simulink model "HallEffect"  (R2024b)
settings: Solver=FixedStepAuto  StartTime=0.0  StopTime=inf  FixedStep=0.01  RelTol=1e-3  EnableMultiTasking=on
libraries: stm32f4xxblockslib x1, simulink x1, dspstat3 x1
settings Model: STM32="{\"AnalogInput\":[{\"ID\":\"untitled:1\"},{\"ID\":\"HallEffect:1\"}]}"  Creator=jirat  LastModifiedBy=jirat
settings OptimizationCC: DefaultParameterBehavior=Inlined  EnhancedBackFolding=on  PassReuseOutputArgsAs=Individual arguments  ZeroExternalMemoryAtStartup=off  ZeroInternalMemoryAtStartup=off  MaxStackSize=512  OptimizeBlockOrder=speed  DifferentSizesBufferReuse=on  OptimizationCustomize=off  EfficientTunableParamExpr=on
settings DebuggingCC: ParameterTunabilityLossMsg=error
settings HardwareCC: ProdBitPerPointer=32  ProdBitPerSizeT=32  ProdBitPerPtrDiffT=32  ProdLargestAtomicInteger=Long  ProdLargestAtomicFloat=Double  ProdWordSize=32  ProdLongLongMode=on  ProdHWDeviceType=ARM Compatible->ARM Cortex-M
settings SFSimCC: MATLABDynamicMemAlloc=off
settings RTWCC: Description=Embedded Coder  SystemTargetFile=ert.tlc  HardwareBoard=STM32G4xx Based  TemplateMakefile=ert_default_tmf  Toolchain=GNU Tools for ARM Embedded Processors
settings CodeAppCC: ForceParamTrailComments=on  IgnoreCustomStorageClasses=off  OperatorAnnotations=on  SimulinkDataObjDesc=on  SFDataObjDesc=on  InsertBlockDesc=on
settings ERTTargetCC: TargetLangStandard=C99 (ISO)  CodeReplacementLibrary=ARM Cortex-M  ExtModeTransport=3  ExtModeStaticAlloc=on  ExtModeStaticAllocSize=2048  ExtModeMexFile=ext_xcp  ExtModeIntrfLevel=Level2 - Open

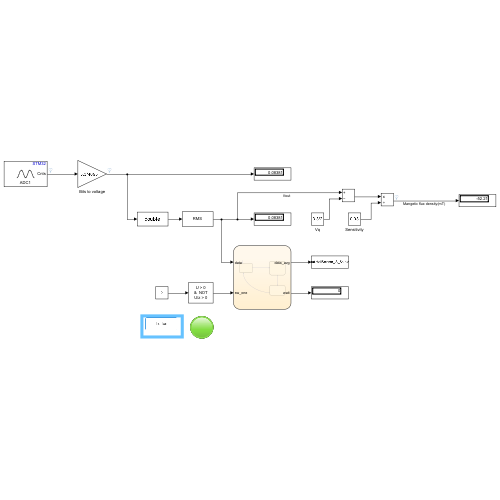
[thumbnail: Simulink's stored preview of the top-level diagram]
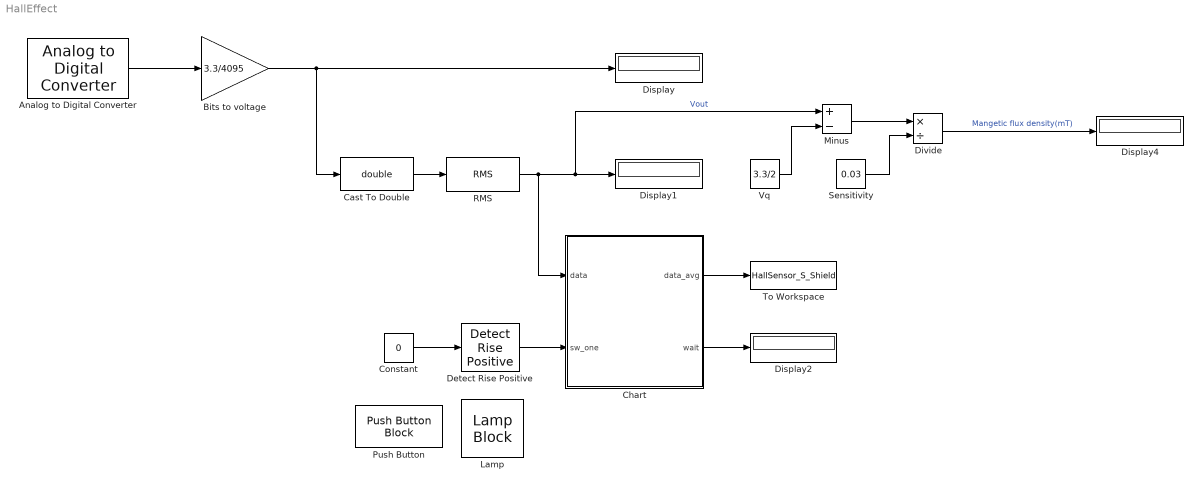
== system HallEffect ==
  Analog to Digital Converter : stm32f4xxblockslib/Analog to Digital Converter  ADCModule=ADC1  ConversionGroup=Regular  TriggerMode=Trigger and read  NumberOfConversions=1  EnableBufferConv=off  BufferLength=1  OutputStatus=off  SampleTime=-1  EnableSimPort=off  hoistedMaskSrc=ECSoC/ECSimCodegen/Analog to Digital Converter
  Bits to voltage : Gain  Gain=3.3/4095
  Cast To Double : DataTypeConversion  OutDataTypeStr=double  SaturateOnIntegerOverflow=off  RndMeth=Floor
  Chart : Stateflow chart  TreatAsAtomicUnit=on
  Constant : Constant  Value=0
  Detect Rise Positive : simulink/Logic and Bit Operations/Detect Rise Positive  vinit=0  OutDataTypeStr=boolean
  Display{,1..2,4} (4 alike) : Display
  Divide : Product  Inputs=*/
  Lamp : LampBlock  LabelPosition=Hide
  Minus : Sum  Inputs=+-
  Push Button : PushButtonBlock  OffValue=0.000000
  RMS : dspstat3/RMS  run=off  directionMode=Each column  dimension=1  InputProcessing=Columns as channels (frame based)  reset_popup=None
  Sensitivity : Constant  Value=0.03
  To Workspace : ToWorkspace  VariableName=HallSensor_S_Shield  SampleTime=-1
      settings: Save2DSignal=2-D array (concatenate along first dimension)
  Vq : Constant  Value=3.3/2
  wires:
  Bits to voltage/1 -> Cast To Double/1, Display/1
  Analog to Digital Converter/1 -> Bits to voltage/1
  RMS/1 -> Minus/1, Display1/1, Chart/1(data)  "Vout"
  Constant/1 -> Detect Rise Positive/1
  Cast To Double/1 -> RMS/1
  Detect Rise Positive/1 -> Chart/2(sw_one)
  Chart/1(data_avg) -> To Workspace/1
  Chart/2(wait) -> Display2/1
  Vq/1 -> Minus/2
  Minus/1 -> Divide/1
  Sensitivity/1 -> Divide/2
  Divide/1 -> Display4/1  "Mangetic flux density(mT)"

== stateflow chart HallEffect/Chart ==
  state wait
    entry :
    time = 0
    back = 0
    wait = 1
    during:
    time = time + 0.01
    if time >= 1
    back = 1
    end
  state Init
    sw_one;
    data;
    back = 0
    wait = 0
  state Action
    data_avg = data
  (default) -> Init
  Init -> wait : [sw_one == 1]
  Action -> Init
  wait -> Action : [back == 1]
  data: data input; sw_one input; data_avg output; time local; wait output; back local
